simulink model "Hw2_ME8352sim"  (R2020b)
settings: Solver=VariableStepAuto  StartTime=0.0  StopTime=t_sim  RelTol=1e-5
values from neighbouring files (symbols this model uses):
  a_ = -1    [Hw2_ME8352.m]
  b_ = 0.03    [Hw2_ME8352.m]
  beta_ = 3    [Hw2_ME8352.m]
  gamma_ = gamma_array(end)    [Hw2_ME8352.m]
  omega_ = 1.2    [Hw2_ME8352.m]
  x_0 = x0_array(i)    [Hw2_ME8352.m]
  xdot_0 = 0    [Hw2_ME8352.m]
undefined symbols (not defined in the file or in its folder): alpha_, g, length_a
libraries: pid_lib x1
settings Model: Creator=dempseca  LastModifiedBy=dempseca

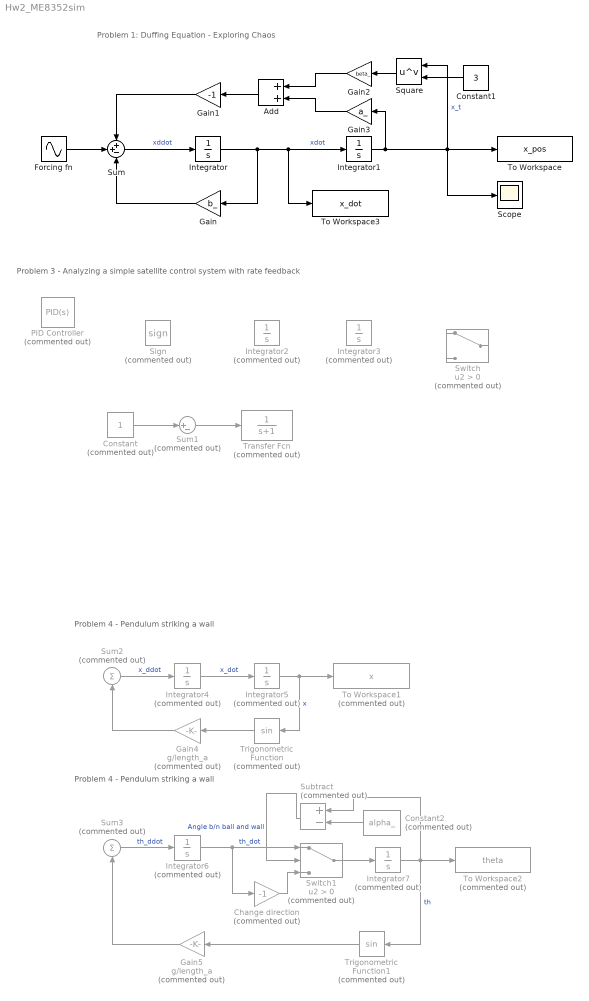
== system Hw2_ME8352sim ==
  note: Problem 4 - Pendulum striking a wall
  note: Problem 3 - Analyzing a simple satellite control system with rate feedback
  note: Problem 1: Duffing Equation - Exploring Chaos
  note: Problem 4 - Pendulum striking a wall
  Add : Sum
  Change direction : Gain  Commented=on  Gain=-1
  Constant : Constant  Commented=on
  Constant1 : Constant  Value=3
  Constant2 : Constant  Commented=on  Value=alpha_
  Forcing fn : Sin  Amplitude=gamma_  Frequency=omega_  Phase=pi/2  SampleTime=0
  Gain : Gain  Gain=b_
  Gain1 : Gain  Gain=-1
  Gain2 : Gain  Gain=beta_
  Gain3 : Gain  Gain=a_
  Gain4 : Gain  Commented=on  Gain=g/length_a
  Gain5 : Gain  Commented=on  Gain=g/length_a
  Integrator : Integrator  InitialCondition=xdot_0
  Integrator1 : Integrator  InitialCondition=x_0
  Integrator{2..7} (6 alike) : Integrator  Commented=on
  PID Controller : pid_lib/PID Controller  Commented=on  Controller=PID  Form=Parallel  TimeDomain=Continuous-time  UseExternalTs=off  SampleTime=-1  IntegratorMethod=Forward Euler  FilterMethod=Forward Euler  ControllerParametersSource=internal  P=1  I=1  D=0  UseFilter=on  N=100  TunerSelectOption=Transfer Function Based (PID Tuner App)  InitialConditionSource=internal  InitialConditionForIntegrator=0  InitialConditionForFilter=0  DifferentiatorICPrevScaledInput=0  ExternalReset=none  TrackingMode=off  Kt=1  LimitOutput=off  SatLimitsSource=internal  UpperSaturationLimit=inf  LowerSaturationLimit=-inf  LinearizeAsGain=on  AntiWindupMode=none  Kb=1  POutMin=[]  POutMax=[]  IOutMin=[]  IOutMax=[]  DOutMin=[]  DOutMax=[]  NOutMin=[]  NOutMax=[]  SumOutMin=[]  SumOutMax=[]  SaturationOutMin=[]  SaturationOutMax=[]  PParamMin=[]  PParamMax=[]  IParamMin=[]  IParamMax=[]  DParamMin=[]  DParamMax=[]  NParamMin=[]  NParamMax=[]  KbParamMin=[]  KbParamMax=[]  KtParamMin=[]  KtParamMax=[]  KbOutMin=[]  KbOutMax=[]  KtOutMin=[]  KtOutMax=[]  IntegratorOutMin=[]  IntegratorOutMax=[]  FilterOutMin=[]  FilterOutMax=[]  SumI1OutMin=[]  SumI1OutMax=[]  SumI2OutMin=[]  SumI2OutMax=[]  SumI3OutMin=[]  SumI3OutMax=[]  SumI4OutMin=[]  SumI4OutMax=[]  SumDOutMin=[]  SumDOutMax=[]  DifferentiatorOutMin=[]  DifferentiatorOutMax=[]  FilterDiffOutCoefMin=[]  FilterDiffOutCoefMax=[]  ReciprocalOutMin=[]  ReciprocalOutMax=[]  SumDenOutMin=[]  SumDenOutMax=[]  SumNumOutMin=[]  SumNumOutMax=[]  DivideOutMin=[]  DivideOutMax=[]  UdiffTsProdOutMin=[]  UdiffTsProdOutMax=[]  NTsProdOutMin=[]  NTsProdOutMax=[]  UintegralTsProdOutMin=[]  UintegralTsProdOutMax=[]  UngainTsProdOutMin=[]  UngainTsProdOutMax=[]  IntegratorContinuousStateAttributes=''  IntegratorStateMustResolveToSignalObject=off  IntegratorRTWStateStorageClass=Auto  FilterContinuousStateAttributes=''  FilterStateMustResolveToSignalObject=off  FilterRTWStateStorageClass=Auto  ParallelPVariant=InternalParameters  IdealPVariant=Disabled  IVariant=InternalParameters  DVariant=InternalParameters  IntegratorVariant=Continuous  SatVariant=Disabled  AWVariant=Passthrough  PCopyVariant=Disabled  TRVariant=Disabled  FdbkBlocksVariant=Forward  IdealPFdbkVariant=Disabled  SatFdbkVariant=Disabled  DerivativeFilterVariant=ContFilter  NVariant=InternalParameters  NCopyVariant=Disabled  FilterICVariant=InternalICsFilter  IntegratorICVariant=InternalICs  ExternalResetVariant=Disabled  TRSumVariant=Passthrough  SumFdbkVariant=Disabled  SumVariant=Sum_PID  TsampFilterVariant=InternalTs  TsampNgainVariant=Passthrough  TsampIntegralVariant=Passthrough  ExternalSaturationOutDataTypeStr=Inherit: Same as second input
  Scope : Scope
  Sign : Signum  Commented=on
  Square : Math  Operator=pow  SaturateOnIntegerOverflow=on
  Subtract : Sum  Commented=on  Inputs=+-
  Sum : Sum  Inputs=++-
  Sum1 : Sum  Commented=on  Inputs=|+-
  Sum2 : Sum  Commented=on  Inputs=|+
  Sum3 : Sum  Commented=on  Inputs=|+
  Switch : Switch  Commented=on  Criteria=u2 > Threshold
  Switch1 : Switch  Commented=on  Criteria=u2 > Threshold
  To Workspace : ToWorkspace  VariableName=x_pos  SaveFormat=Timeseries  SampleTime=-1
  To Workspace1 : ToWorkspace  Commented=on  VariableName=x  SaveFormat=Timeseries  SampleTime=-1
  To Workspace2 : ToWorkspace  Commented=on  VariableName=theta  SaveFormat=Timeseries  SampleTime=-1
  To Workspace3 : ToWorkspace  VariableName=x_dot  SaveFormat=Timeseries  SampleTime=-1
  Transfer Fcn : TransferFcn  Commented=on  Denominator=[1 1]
  Trigonometric Function : Trigonometry  Commented=on
  Trigonometric Function1 : Trigonometry  Commented=on
  wires:
  Integrator/1 -> Gain/1, To Workspace3/1, Integrator1/1  "xdot"
  Integrator1/1 -> Gain3/1, Scope/1, Square/1, To Workspace/1  "x_t"
  Sum/1 -> Integrator/1  "xddot"
  Gain/1 -> Sum/3
  Gain1/1 -> Sum/1
  Add/1 -> Gain1/1
  Constant1/1 -> Square/2
  Gain3/1 -> Add/2
  Gain2/1 -> Add/1
  Square/1 -> Gain2/1
  Forcing fn/1 -> Sum/2
  Constant/1 -> Sum1/1
  Sum1/1 -> Transfer Fcn/1
  Integrator4/1 -> Integrator5/1  "x_dot"
  Integrator5/1 -> Trigonometric Function/1, To Workspace1/1  "x"
  Sum2/1 -> Integrator4/1  "x_ddot"
  Trigonometric Function/1 -> Gain4/1
  Gain4/1 -> Sum2/1
  Sum3/1 -> Integrator6/1  "th_ddot"
  Integrator7/1 -> Subtract/1, Trigonometric Function1/1, To Workspace2/1  "th"
  Trigonometric Function1/1 -> Gain5/1
  Gain5/1 -> Sum3/1
  Integrator6/1 -> Change direction/1, Switch1/1  "th_dot"
  Switch1/1 -> Integrator7/1
  Change direction/1 -> Switch1/3
  Constant2/1 -> Subtract/2
  Subtract/1 -> Switch1/2  "Angle b/n ball and wall"
